simulink model "labwork_01"  (R2021a)
settings: Solver=VariableStepAuto  StartTime=0.0  StopTime=10.0  RelTol=1e-3
settings Model: Creator=alamg  LastModifiedBy=alamg

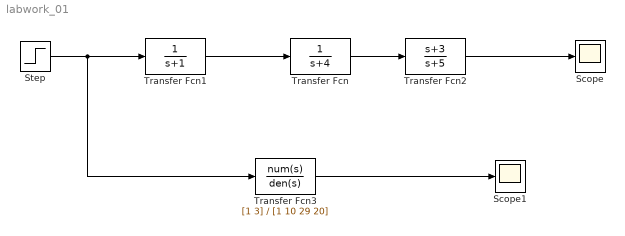
== system labwork_01 ==
  Scope : Scope
  Scope1 : Scope
  Step : Step  SampleTime=0
  Transfer Fcn : TransferFcn  Denominator=[1 4]
  Transfer Fcn1 : TransferFcn  Denominator=[1 1]
  Transfer Fcn2 : TransferFcn  Numerator=[1 3]  Denominator=[1 5]
  Transfer Fcn3 : TransferFcn  Numerator=[1 3]  Denominator=[1 10 29 20]
  wires:
  Transfer Fcn1/1 -> Transfer Fcn/1
  Transfer Fcn/1 -> Transfer Fcn2/1
  Transfer Fcn2/1 -> Scope/1
  Transfer Fcn3/1 -> Scope1/1
  Step/1 -> Transfer Fcn3/1, Transfer Fcn1/1
